simulink model "pv"  (R2018a)
settings: Solver=ode4  StartTime=0.0  StopTime=10.0  FixedStep=1e-4  RelTol=1e-3
InitFcn:
  | SimulinkInit
settings Model: Creator=carma  LastModifiedBy=AndrewB
settings OptimizationCC: DefaultParameterBehavior=Inlined  EnhancedBackFolding=on  PassReuseOutputArgsAs=Individual arguments  OptimizeBlockOrder=speed  DifferentSizesBufferReuse=on  OptimizationCustomize=off
settings DebuggingCC: ParameterTunabilityLossMsg=error
settings SFSimCC: MATLABDynamicMemAlloc=off
settings RTWCC: SystemTargetFile=ert.tlc  TemplateMakefile=ert_default_tmf  GenerateReport=on  IncludeHyperlinkInReport=on  LaunchReport=on  GenerateTraceInfo=on  GenerateTraceReport=on  GenerateTraceReportSl=on  GenerateTraceReportSf=on  GenerateTraceReportEml=on
settings CodeAppCC: ForceParamTrailComments=on  IgnoreCustomStorageClasses=off  OperatorAnnotations=on  SimulinkDataObjDesc=on  SFDataObjDesc=on  InsertBlockDesc=on
settings ERTTargetCC: TargetLangStandard=C99 (ISO)  GenerateSampleERTMain=on  SupportContinuousTime=on  InlinedParameterPlacement=NonHierarchical  ERTCustomFileTemplate=example_file_process.tlc

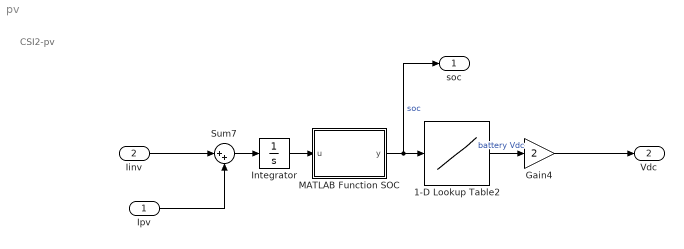
== system pv ==
  note: CSI2-pv
  Ipv : Inport
  Iinv : Inport  Port=2
  1-D Lookup Table2 : Lookup_n-D  NumberOfTableDimensions=1  BreakpointsForDimension1=[0 10 20 30 40 50 70 80 100]  Table=[0 10 200 500 800 1000 1140 1150 1200]  InternalRulePriority=Speed  RndMeth=Simplest  InputSameDT=on
  Gain4 : Gain  Gain=2
  Integrator : Integrator  LimitOutput=on  UpperSaturationLimit=1  LowerSaturationLimit=0
  "MATLAB Function SOC " : MATLAB Function  TreatAsAtomicUnit=on
  Sum7 : Sum  Inputs=|++
  soc : Outport
  Vdc : Outport  Port=2
  wires:
  Gain4/1 -> Vdc/1
  Ipv/1 -> Sum7/2
  "MATLAB Function SOC "/1(y) -> soc/1, 1-D Lookup Table2/1  "soc"
  1-D Lookup Table2/1 -> Gain4/1  "battery Vdc"
  Integrator/1 -> "MATLAB Function SOC "/1(u)
  Sum7/1 -> Integrator/1
  Iinv/1 -> Sum7/1

== matlab function pv/MATLAB Function SOC  ==
  data: u input; y output
function y = fcn(u)

y = -0.03536*u+100;
